simulink model "b_node"  (R2012b)
settings: Solver=FixedStepDiscrete  SolverMode=SingleTasking  StartTime=0.0  StopTime=inf  RelTol=1e-3
model workspace (MAT data in the model file):
  lambda = Simulink.Parameter
  lambda.DataType = 'auto'
libraries: simulink x2
settings Model: Creator=andreas  LastModifiedBy=andreas
settings DataIOCC: SaveOutput=off  SignalLogging=off  SaveTime=off
settings OptimizationCC: InlineParams=on
settings DebuggingCC: AlgebraicLoopMsg=error  SingleTaskRateTransMsg=error
settings ModelReferenceCC: UpdateModelReferenceTargets=IfOutOfDate

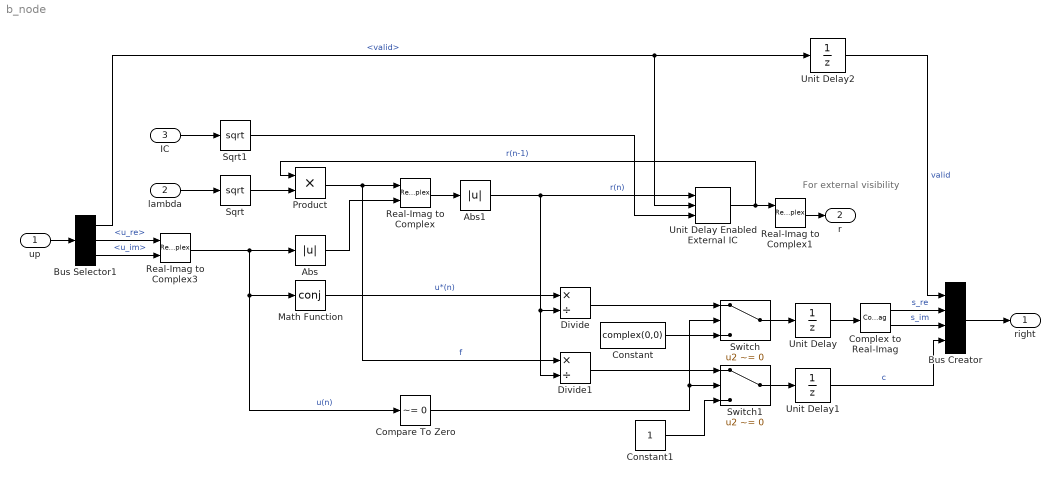
== system b_node ==
  note: For external
      | visibility
  up : Inport  OutDataTypeStr=Bus: vbus
  lambda : Inport  Port=2
  IC : Inport  Port=3
  Abs : Abs
  Abs1 : Abs
  Bus Creator : BusCreator
  Bus Selector1 : BusSelector  OutputSignals=valid,u_re,u_im
  Compare To Zero : simulink/Logic and Bit Operations/Compare To Zero  relop=~=  OutDataTypeStr=boolean
  Complex to Real-Imag : ComplexToRealImag
  Constant : Constant  Value=complex(0,0)
  Constant1 : Constant
  Divide : Product  Inputs=*/
  Divide1 : Product  Inputs=*/
  Math Function : Math  Operator=conj  SaturateOnIntegerOverflow=on
  Product : Product  RndMeth=Zero
  Real-Imag to Complex : RealImagToComplex
  Real-Imag to Complex1 : RealImagToComplex
  Real-Imag to Complex3 : RealImagToComplex
  Sqrt : Sqrt  SaturateOnIntegerOverflow=on
  Sqrt1 : Sqrt  SaturateOnIntegerOverflow=on
  Switch : Switch  Criteria=u2 ~= 0
  Switch1 : Switch  Criteria=u2 ~= 0
  Unit Delay : UnitDelay  SampleTime=-1
  Unit Delay Enabled External IC : simulink/Additional Math & Discrete/Additional Discrete/Unit Delay Enabled External IC  tsamp=-1
  Unit Delay1 : UnitDelay  SampleTime=-1
  Unit Delay2 : UnitDelay  SampleTime=-1
  right : Outport  OutDataTypeStr=Bus: hbus
      settings: SignalType=complex
  r : Outport  Port=2
      settings: SignalType=complex
  wires:
  Sqrt/1 -> Product/2
  Real-Imag to Complex3/1 -> Compare To Zero/1, Math Function/1, Abs/1  "u(n)"
  Abs1/1 -> Divide1/2, Divide/2, Unit Delay Enabled External IC/1  "r(n)"
  Unit Delay Enabled External IC/1 -> Real-Imag to Complex1/1, Product/1  "r(n-1)"
  Abs/1 -> Real-Imag to Complex/2
  Product/1 -> Divide1/1, Real-Imag to Complex/1  "f"
  Real-Imag to Complex/1 -> Abs1/1
  Unit Delay1/1 -> Bus Creator/4  "c"
  Math Function/1 -> Divide/1  "u*(n)"
  lambda/1 -> Sqrt/1
  Real-Imag to Complex1/1 -> r/1
  IC/1 -> Sqrt1/1
  Sqrt1/1 -> Unit Delay Enabled External IC/3
  Divide/1 -> Switch/1
  Switch/1 -> Unit Delay/1
  Divide1/1 -> Switch1/1
  Switch1/1 -> Unit Delay1/1
  Compare To Zero/1 -> Switch1/2, Switch/2
  Constant/1 -> Switch/3
  Constant1/1 -> Switch1/3
  Bus Selector1/1 -> Unit Delay Enabled External IC/2, Unit Delay2/1  "<valid>"
  Bus Selector1/2 -> Real-Imag to Complex3/1  "<u_re>"
  Bus Selector1/3 -> Real-Imag to Complex3/2  "<u_im>"
  up/1 -> Bus Selector1/1
  Unit Delay/1 -> Complex to Real-Imag/1
  Complex to Real-Imag/1 -> Bus Creator/2  "s_re"
  Complex to Real-Imag/2 -> Bus Creator/3  "s_im"
  Bus Creator/1 -> right/1
  Unit Delay2/1 -> Bus Creator/1  "valid"
